simulink model "sim_tracking_1"  (R2023b)
settings: Solver=ode23  StartTime=0.0  StopTime=Tfin  RelTol=1e-3  EnableMultiTasking=on
values from neighbouring files (symbols this model uses):
  hr = diag(ll/2)*hr    [main_regulation.m]    (also in main_tracking_1.m; simulation_dyn_kin.m = diag([1 1.5 3]/2)*hr)
  IJ = inv(J)    [main_regulation.m]    (also in main_tracking_1.m; main_tracking_2.m)
  J = diag([10 9 12]*1e3)    [main_regulation.m]    (also in main_tracking_1.m; main_tracking_2.m = diag(J0))
  q0 = [0.6853;0.6953;0.1531;0.1531]    [main_regulation.m]    (also in main_tracking_1.m = [cos(th0/2);0;sin(th0/2);0]; main_tracking_2.m = [1;0;0;0]; simulation_dyn_kin.m = [1;0;0;0])
  qr = [1;0;0;0]    [main_regulation.m]    (also in main_tracking_1.m = [cos(th/2);0;sin(th/2);0])
  w0 = [0.53;0.53;0.053]    [main_regulation.m]    (also in main_tracking_1.m = [0;0;0]; main_tracking_2.m = [0;0;0]; simulation_dyn_kin.m = [0.01;0;1]; simulation_euler.m = [0.25;0;0.63])
  wr = [0;0;0]    [main_tracking_1.m]    (also in main_tracking_2.m = [0.3;0;0])
undefined symbols (not defined in the file or in its folder): animation_rot, qua2euler
libraries: vrlib x1
settings Model: Creator=carlonovara  LastModifiedBy=carlonovara
settings SolverCC: AlgebraicLoopSolver=TrustRegion
settings DataIOCC: ReturnWorkspaceOutputs=off
settings OptimizationCC: LifeSpan=inf
settings DebuggingCC: UnconnectedInputMsg=warning  UnconnectedOutputMsg=warning  UnconnectedLineMsg=warning  SFUnexpectedBacktrackingDiag=warning  SFNoUnconditionalDefaultTransitionDiag=warning  SFExecutionAtInitializationDiag=none  ArithmeticOperatorsInVariantConditions=warning
settings ModelReferenceCC: EnableRefExpFcnMdlSchedulingChecks=on
settings SFSimCC: SimUseLocalCustomCode=off  CustomCodeUndefinedFunction=UseInterfaceOnly
settings RTWCC: RTWUseLocalCustomCode=off
settings CodeAppCC: StateflowObjectComments=on
settings GRTTargetCC: TargetLangStandard=C89/C90 (ANSI)
settings ConfigComp: CovMetricSettings=dw  CovSaveCumulativeToWorkspaceVar=on  CovSaveSingleToWorkspaceVar=on  CovExternalEMLEnable=off

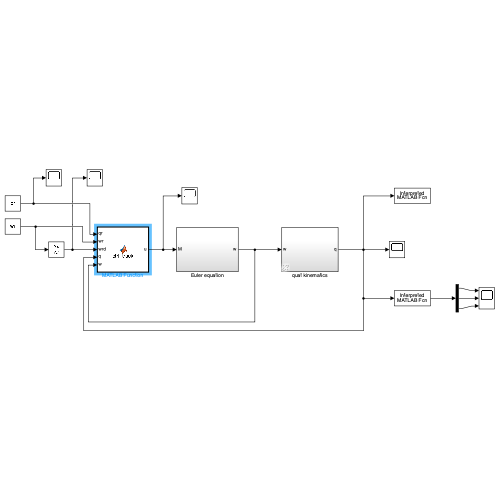
[thumbnail: Simulink's stored preview of the top-level diagram]
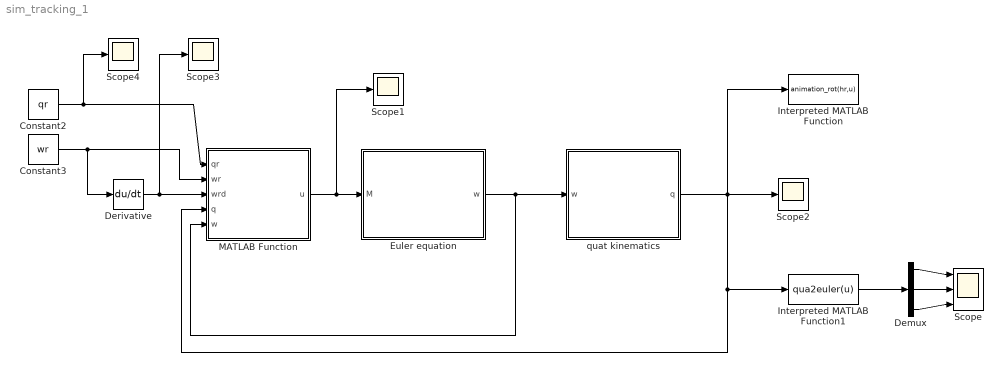
== system sim_tracking_1 ==
  Constant2 : Constant  Value=qr
  Constant3 : Constant  Value=wr
  Demux : Demux  Outputs=3
  Derivative : Derivative  CoefficientInTFapproximation=50
  Euler equation : Subsystem
  Interpreted MATLAB Function : MATLABFcn  MATLABFcn=animation_rot(hr,u)  OutputDimensions=0
  Interpreted MATLAB Function1 : MATLABFcn  MATLABFcn=qua2euler(u)
  MATLAB Function : MATLAB Function  TreatAsAtomicUnit=on
  Scope : Scope  NumInputPorts=3
  Scope{1..4} (4 alike) : Scope
  quat kinematics : Subsystem  AncestorBlock=lib_rotations_2014/quat kinematics
  wires:
  MATLAB Function/1(u) -> Scope1/1, Euler equation/1(M)
  Euler equation/1(w) -> quat kinematics/1(w), MATLAB Function/5(w)
  Interpreted MATLAB Function1/1 -> Demux/1
  Demux/1 -> Scope/1
  Demux/2 -> Scope/2
  Demux/3 -> Scope/3
  Constant2/1 -> Scope4/1, MATLAB Function/1(qr)
  quat kinematics/1(q) -> Interpreted MATLAB Function/1, Scope2/1, MATLAB Function/4(q), Interpreted MATLAB Function1/1
  Constant3/1 -> Derivative/1, MATLAB Function/2(wr)
  Derivative/1 -> Scope3/1, MATLAB Function/3(wrd)

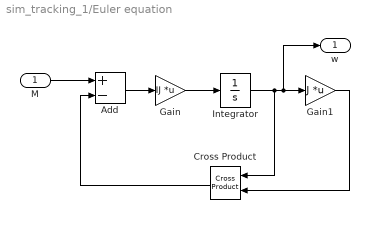
== system sim_tracking_1/Euler equation ==
  M : Inport
  Add : Sum  Inputs=+-
  Cross Product : vrlib/Utilities/Cross Product
  Gain : Gain  Gain=IJ  Multiplication=Matrix(K*u)
  Gain1 : Gain  Gain=J  Multiplication=Matrix(K*u)
  Integrator : Integrator  InitialCondition=w0
  w : Outport  VectorParamsAs1DForOutWhenUnconnected=off
  wires:
  M/1 -> Add/1
  Integrator/1 -> Cross Product/1, w/1, Gain1/1
  Gain/1 -> Integrator/1
  Gain1/1 -> Cross Product/2
  Add/1 -> Gain/1
  Cross Product/1 -> Add/2

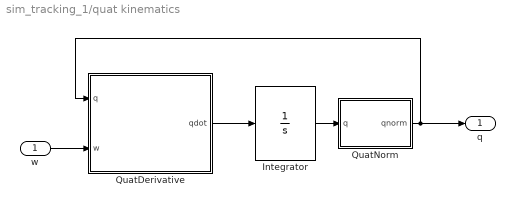
== system sim_tracking_1/quat kinematics ==
  w : Inport  PortDimensions=3
  Integrator : Integrator  InitialCondition=q0
  QuatDerivative : MATLAB Function  TreatAsAtomicUnit=on
  QuatNorm : MATLAB Function  TreatAsAtomicUnit=on
  q : Outport  PortDimensions=4  VectorParamsAs1DForOutWhenUnconnected=off
  wires:
  w/1 -> QuatDerivative/2(w)
  QuatDerivative/1(qdot) -> Integrator/1
  QuatNorm/1(qnorm) -> QuatDerivative/1(q), q/1
  Integrator/1 -> QuatNorm/1(q)

== matlab function sim_tracking_1/quat kinematics/QuatDerivative ==
  data: q input; qdot output; w input
function qdot= QuatDerivative(q,w)
%#codegen
omegaq=[0; w];
Q=[q(1) -q(2) -q(3) -q(4);
    q(2) q(1) -q(4) q(3);
    q(3) q(4) q(1) -q(2);
    q(4) -q(3) q(2) q(1)];
qdot=Q*omegaq/2;

== matlab function sim_tracking_1/MATLAB Function ==
  data: qr input; wr input; wrd input; q input; u output; w input
function u = ctrl_track(qr,wr,wrd,q,w)
%#codegen

J=diag([10 9 12]*1e3);

u=zeros(3,1);

qs=[q(1);-q(2:4)];
dq=quatprod(qs,qr);
dw=wr-w;

% Proportional-Derivative controller
% kp=2;
% kd=200;
% u=kp*dq(2:4)+kd*dw;
% %u=kp*sign(dq(1))*dq(2:4)+kd*dw;

% Sliding Mode Control - version 1
k2=0.1;
k1=50;
us=J*(wrd+k2/2*(dq(1)*dw+crossprod(dq(2:4),wr+w)))+crossprod(w,J*w);
s=dw+k2*dq(2:4);
u=us+k1*tanh(s);

% Sliding Mode Control - version 2
% k2=0.1;
% k1=50;
% us=J*(wrd+k2/2*(abs(dq(1))*dw+sign(q(1))*crossprod(dq(2:4),wr+w)))+crossprod(w,J*w);
% s=dw+k2*sign(q(1))*dq(2:4);
% u=us+k1*tanh(s);

end

== matlab function sim_tracking_1/quat kinematics/QuatNorm ==
  data: q input; qnorm output
function qnorm = QuatNorm(q)
%#codegen
qnorm=zeros(4,1);
q2=sqrt(q'*q);
qnorm=q/q2;
